simulink model "main_SLDV_2_2020"  (R2020b)
settings: Solver=FixedStepDiscrete  StartTime=0.0  StopTime=20.0  FixedStep=1  RelTol=1e-3
libraries: sldvlib x13, simulink x1
settings Model: Creator=ayj  LastModifiedBy=adije
settings DebuggingCC: UnconnectedInputMsg=none  UnconnectedOutputMsg=none  UnconnectedLineMsg=none  SFMachineParentedDataDiag=error
settings ConfigComp: DVMode=PropertyProving  DVTestSuiteOptimization=Auto  DVDetectOutOfBounds=on  DVProvingStrategy=FindViolation  DVMaxViolationSteps=12

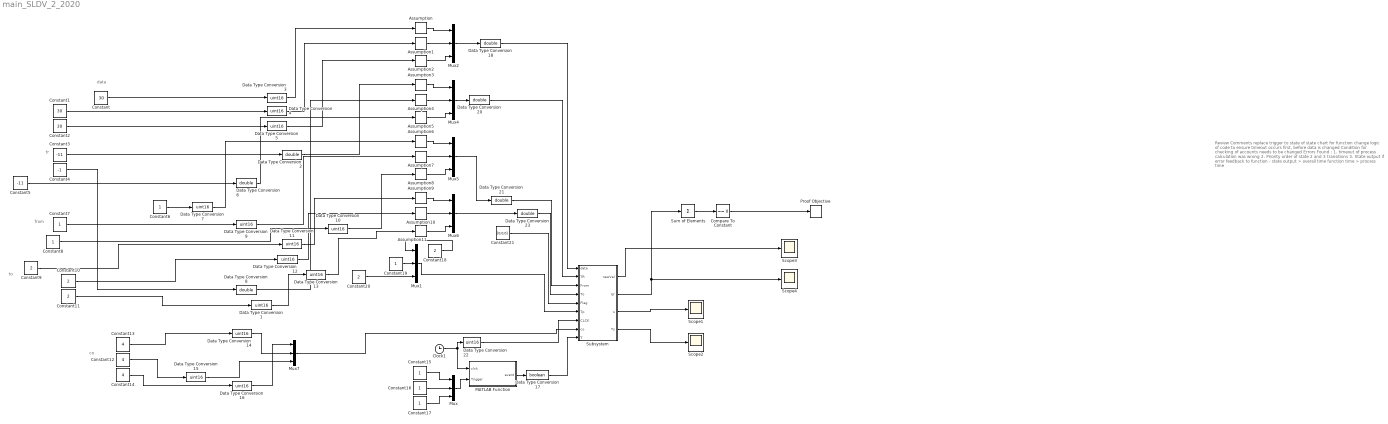
== system main_SLDV_2_2020 ==
  note: data
  note: tr
  note: from
  note: to
  note: co
  note: Review Comments
      | replace trigger to state of state chart for function
      | change logic of code to ensure timeout occurs first, before data is changed
      | Condition for checking of accounts needs to be changed
      |
      | Errors Found :
      | 1. timeout of process calculation was wrong
      | 2. Priority order of state 2 and 3 transitions
      | 3. State output if error feedback to function - state output > overall time
      | function time > process time
  Assumption : sldvlib/Objectives and Constraints/Assumption  enabled=on  customAVTBlockType=Assumption  intervals={30, 31, 32}  initial=off  dispValues=on  outEnabled=on
      settings: AttributesFormatString=%<intervals>  SourceProductBaseCode=SL
  Assumption1 : sldvlib/Objectives and Constraints/Assumption  enabled=on  customAVTBlockType=Assumption  intervals={30, 31, 32}  initial=off  dispValues=on  outEnabled=on
      settings: AttributesFormatString=%<intervals>  SourceProductBaseCode=SL
  Assumption{6..11} (6 alike) : sldvlib/Objectives and Constraints/Assumption  enabled=on  customAVTBlockType=Assumption  intervals={1,2,3}  initial=off  dispValues=on  outEnabled=on
      settings: AttributesFormatString=%<intervals>  SourceProductBaseCode=SL
  Assumption2 : sldvlib/Objectives and Constraints/Assumption  enabled=on  customAVTBlockType=Assumption  intervals={30, 31, 32}  initial=off  dispValues=on  outEnabled=on
      settings: AttributesFormatString=%<intervals>  SourceProductBaseCode=SL
  Assumption3 : sldvlib/Objectives and Constraints/Assumption  enabled=on  customAVTBlockType=Assumption  intervals={-10,+10,0, -11}  initial=off  dispValues=on  outEnabled=on
      settings: AttributesFormatString=%<intervals>  SourceProductBaseCode=SL
  Assumption4 : sldvlib/Objectives and Constraints/Assumption  enabled=on  customAVTBlockType=Assumption  intervals={-10,+10,0, -11}  initial=off  dispValues=on  outEnabled=on
      settings: AttributesFormatString=%<intervals>  SourceProductBaseCode=SL
  Assumption5 : sldvlib/Objectives and Constraints/Assumption  enabled=on  customAVTBlockType=Assumption  intervals={-10,+10,0, -11}  initial=off  dispValues=on  outEnabled=on
      settings: AttributesFormatString=%<intervals>  SourceProductBaseCode=SL
  Clock1 : Clock
  Compare To Constant : simulink/Logic and Bit Operations/Compare To Constant  relop===  const=0  OutDataTypeStr=boolean
  Constant : Constant  Value=30
  Constant1 : Constant  Value=30
  Constant{9..11,18,20} (5 alike) : Constant  Value=2
  Constant12 : Constant  Value=4
  Constant13 : Constant  Value=4
  Constant14 : Constant  Value=4
  Constant{6..8,15..17,19} (7 alike) : Constant
  Constant2 : Constant  Value=30
  Constant21 : Constant  Value=[0,0,0]
  Constant3 : Constant  Value=-11
  Constant4 : Constant  Value=-1
  Constant5 : Constant  Value=-11
  Data Type Conversion{1,3..5,7,9..16,22} (14 alike) : DataTypeConversion  OutDataTypeStr=uint16  RndMeth=Round
  Data Type Conversion17 : DataTypeConversion  OutDataTypeStr=boolean  RndMeth=Round
  Data Type Conversion{2,6,8,18,20..21,23} (7 alike) : DataTypeConversion  OutDataTypeStr=double  RndMeth=Round
  MATLAB Function : MATLAB Function  TreatAsAtomicUnit=on
  Mux{,1..2,4..7} (7 alike) : Mux  Inputs=3
  Proof Objective : sldvlib/Objectives and Constraints/Proof Objective  enabled=on  customAVTBlockType=Proof Objective  intervals=true  dispValues=on  outEnabled=off  enableStopSim=off
      settings: AttributesFormatString=%<intervals>  SourceProductBaseCode=SL
  Scope{1..4} (4 alike) : Scope
  Subsystem : Subsystem
  Sum of Elements : Sum  Inputs=+
  wires:
  Constant/1 -> Data Type Conversion3/1
  Constant1/1 -> Data Type Conversion4/1
  Constant2/1 -> Data Type Conversion5/1
  Constant3/1 -> Data Type Conversion2/1
  Constant6/1 -> Data Type Conversion7/1
  Constant7/1 -> Data Type Conversion9/1
  Constant8/1 -> Data Type Conversion10/1
  Constant9/1 -> Data Type Conversion11/1
  Constant10/1 -> Data Type Conversion12/1
  Constant11/1 -> Data Type Conversion1/1
  Constant4/1 -> Data Type Conversion8/1
  Constant5/1 -> Data Type Conversion6/1
  Constant13/1 -> Data Type Conversion14/1
  Constant12/1 -> Data Type Conversion15/1
  Constant14/1 -> Data Type Conversion16/1
  Data Type Conversion1/1 -> Data Type Conversion13/1
  Constant18/1 -> Mux1/1
  Constant20/1 -> Mux1/3
  Assumption4/1 -> Mux4/2
  Assumption7/1 -> Mux5/2
  Sum of Elements/1 -> Compare To Constant/1
  Data Type Conversion12/1 -> Assumption10/1
  Assumption/1 -> Mux2/1
  Mux6/1 -> Data Type Conversion23/1
  Assumption6/1 -> Mux5/1
  Assumption3/1 -> Mux4/1
  Data Type Conversion8/1 -> Assumption4/1
  Data Type Conversion9/1 -> Assumption7/1
  Assumption11/1 -> Mux6/3
  Data Type Conversion13/1 -> Assumption11/1
  Assumption1/1 -> Mux2/2
  Constant17/1 -> Mux/3
  Data Type Conversion11/1 -> Assumption9/1
  Data Type Conversion3/1 -> Assumption/1
  Data Type Conversion4/1 -> Assumption1/1
  Data Type Conversion2/1 -> Assumption3/1
  Mux5/1 -> Data Type Conversion21/1
  Constant15/1 -> Mux/1
  Compare To Constant/1 -> Proof Objective/1
  Mux2/1 -> Data Type Conversion18/1
  Assumption8/1 -> Mux5/3
  Data Type Conversion5/1 -> Assumption2/1
  Assumption9/1 -> Mux6/1
  MATLAB Function/1(event) -> Data Type Conversion17/1
  Data Type Conversion10/1 -> Assumption8/1
  Assumption10/1 -> Mux6/2
  Mux4/1 -> Data Type Conversion20/1
  Constant16/1 -> Mux/2
  Constant19/1 -> Mux1/2
  Assumption2/1 -> Mux2/3
  Assumption5/1 -> Mux4/3
  Data Type Conversion7/1 -> Assumption6/1
  Mux/1 -> MATLAB Function/2(Trigger)
  Clock1/1 -> Data Type Conversion22/1, MATLAB Function/1(clck)
  Data Type Conversion6/1 -> Assumption5/1
  Data Type Conversion16/1 -> Mux7/1
  Data Type Conversion14/1 -> Mux7/2
  Data Type Conversion15/1 -> Mux7/3
  Subsystem/2(Er) -> Sum of Elements/1, Scope4/1
  Data Type Conversion18/1 -> Subsystem/1(data)
  Data Type Conversion20/1 -> Subsystem/2(TR)
  Data Type Conversion21/1 -> Subsystem/3(From)
  Data Type Conversion23/1 -> Subsystem/4(To)
  Constant21/1 -> Subsystem/5(Flag)
  Mux1/1 -> Subsystem/6(Tp)
  Data Type Conversion22/1 -> Subsystem/7(CLCK)
  Mux7/1 -> Subsystem/8(co)
  Data Type Conversion17/1 -> Subsystem/9(T)
  Subsystem/1(newVal) -> Scope3/1
  Subsystem/3(s) -> Scope1/1
  Subsystem/4(Ts) -> Scope2/1

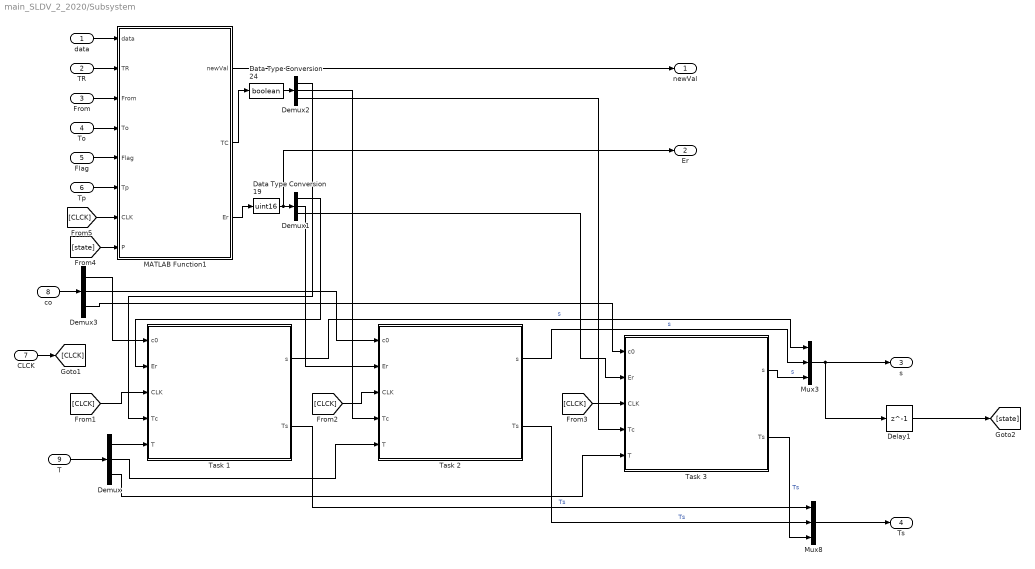
== system main_SLDV_2_2020/Subsystem ==
  data : Inport
  TR : Inport  Port=2
  From : Inport  Port=3
  To : Inport  Port=4
  Flag : Inport  Port=5
  Tp : Inport  Port=6
  CLCK : Inport  Port=7
  co : Inport  Port=8
  T : Inport  Port=9
  Data Type Conversion19 : DataTypeConversion  OutDataTypeStr=uint16  RndMeth=Round
  Data Type Conversion24 : DataTypeConversion  OutDataTypeStr=boolean  RndMeth=Round
  Delay1 : Delay  DelayLength=1
  Demux{,1..3} (4 alike) : Demux  Outputs=3
  MATLAB Function1 : MATLAB Function  TreatAsAtomicUnit=on
  Mux3 : Mux  Inputs=3
  Mux8 : Mux  Inputs=3
  Task 1 : Stateflow chart  TreatAsAtomicUnit=on
  Task 2 : Stateflow chart  TreatAsAtomicUnit=on
  Task 3 : Stateflow chart  TreatAsAtomicUnit=on
  newVal : Outport
  Er : Outport  Port=2
  s : Outport  Port=3
  Ts : Outport  Port=4
  wires:
  data/1 -> MATLAB Function1/1(data)
  Demux/2 -> Task 2/5(T)
  Demux1/2 -> Task 2/2(Er)
  Mux3/1 -> Delay1/1, s/1
  MATLAB Function1/1(newVal) -> newVal/1
  Demux1/3 -> Task 3/2(Er)
  [CLCK] -> MATLAB Function1/7(CLK)
  Task 2/1(s) -> Mux3/2  "s"
  Mux8/1 -> Ts/1
  Demux3/2 -> Task 2/1(c0)
  [CLCK] -> Task 3/3(CLK)
  Data Type Conversion19/1 -> Er/1, Demux1/1
  Task 1/1(s) -> Mux3/1  "s"
  To/1 -> MATLAB Function1/4(To)
  Demux2/1 -> Task 1/4(Tc)
  [CLCK] -> Task 1/3(CLK)
  Demux2/3 -> Task 3/4(Tc)
  Demux/1 -> Task 1/5(T)
  [CLCK] -> Task 2/3(CLK)
  Flag/1 -> MATLAB Function1/5(Flag)
  Demux3/1 -> Task 1/1(c0)
  Demux3/3 -> Task 3/1(c0)
  Demux2/2 -> Task 2/4(Tc)
  Task 3/2(Ts) -> Mux8/3  "Ts"
  Delay1/1 -> [state]
  Demux/3 -> Task 3/5(T)
  MATLAB Function1/3(Er) -> Data Type Conversion19/1
  MATLAB Function1/2(TC) -> Data Type Conversion24/1
  co/1 -> Demux3/1
  Demux1/1 -> Task 1/2(Er)
  Task 3/1(s) -> Mux3/3  "s"
  Tp/1 -> MATLAB Function1/6(Tp)
  Task 2/2(Ts) -> Mux8/2  "Ts"
  From/1 -> MATLAB Function1/3(From)
  CLCK/1 -> [CLCK]
  Task 1/2(Ts) -> Mux8/1  "Ts"
  [state] -> MATLAB Function1/8(P)
  Data Type Conversion24/1 -> Demux2/1
  T/1 -> Demux/1
  TR/1 -> MATLAB Function1/2(TR)

== stateflow chart main_SLDV_2_2020/Subsystem/Task 3 ==
  state Transact
    en:
    s = 1
    Ts = CLK
    du:
    c = c+1
  state Idle
    en:
    c = 0
    s = 0
    Ts = 0
  state Error
    en:
    s = 2
  state Error1
    en:
    s = 3
  Transact -> Error [order 2] : [c>=c0 || Er > 0]
  (default) -> Idle
  Idle -> Transact : [T==1]
  Transact -> Error1 [order 1] : [Tc == 1]
  Error -> Error1
  Error1 -> Idle
  data: c0 input uint16; Er input uint16; CLK input uint16; s output uint16; c local uint16; Ts output uint16; Tc input boolean; T input boolean

== matlab function main_SLDV_2_2020/Subsystem/MATLAB Function1 ==
  data: newVal output; data input double; TR input double; From input double; TC output; To input double; Flag input; Tp input; CLK input; P input; Er output
function [newVal, TC, Er] = fcn(data, TR, From, To, Flag, Tp, CLK, P)
persistent d
persistent f
persistent TC1
persistent Er1
persistent timeo
persistent init
persistent From1
persistent To1
persistent TR1
if(isempty(From1))
    From1 = [1;1;1];
end
if(isempty(To1))
    To1 = [1;1;1];
end
if(isempty(TR1))
    TR1 = [1;1;1];
end
if(isempty(d))
    d = [0;0;0];
end
if(isempty(init))
    init = 0;
end
if(isempty(f))
    f = [0;0;0];
end
if(isempty(TC1))
    TC1 = [0;0;0];
end
if(isempty(Er1))
    Er1 = [0;0;0];
end
if(isempty(timeo))
    timeo = [10,10,10];
end
if(init == 0)
    From1 = From;
    To1 = To;
    TR1 = TR;
    d = data;
    init = 1;
    f = Flag;
end


for i = 1:3
    if P(i) == 1
        if (f(From1(i)) == 0 && f(To1(i)) == 0)
            f(From1(i)) = 1;
            f(To1(i)) = 1;
            timeo(i) = CLK + Tp(i);
            if(d(From1(i)) + TR1(i) < 0 || d(To1(i)) - TR1(i) < 0)
                Er1(i) = 2;
                timeo(i) = 0;
            end
        end
        if CLK >= timeo(i)
            if(Er1(i) ~= 2)
                d(From1(i)) = d(From1(i)) + TR1(i);
                d(To1(i)) = d(To1(i)) - TR1(i);
                TC1(i) = 1;
            end
            f(From1(i)) = 0;
            f(To1(i)) = 0;
        end
    elseif P(i) == 2
        Er1(i) = 1;
    end
end

TC = TC1;
Er = Er1;
newVal = d;

== stateflow chart main_SLDV_2_2020/Subsystem/Task 2 ==
  state Transact
    en:
    s = 1
    Ts = CLK
    du:
    c = c+1
  state Idle
    en:
    c = 0
    s = 0
    Ts = 0
  state Error
    en:
    s = 2
  state Error1
    en:
    s = 3
  Transact -> Error [order 2] : [c>=c0 || Er > 0]
  Idle -> Transact : [T==1]
  (default) -> Idle
  Transact -> Error1 [order 1] : [Tc == 1]
  Error -> Error1
  Error1 -> Idle
  data: c0 input uint16; Er input uint16; CLK input uint16; s output uint16; c local uint16; Ts output uint16; Tc input boolean; T input boolean

== matlab function main_SLDV_2_2020/MATLAB Function ==
  data: clck input; event output; Trigger input
function event = fcn(clck, Trigger)
    event = clck==Trigger;

== stateflow chart main_SLDV_2_2020/Subsystem/Task 1 ==
  state Transact
    en:
    s = 1
    Ts = CLK
    du:
    c = c+1
  state Idle
    en:
    c = 0
    s = 0
    Ts = 0
  state Error
    en:
    s = 2
  state Error1
    en:
    s = 3
  Transact -> Error [order 2] : [c>=c0 || Er > 0]
  (default) -> Idle
  Idle -> Transact : [T==1]
  Transact -> Error1 [order 1] : [Tc == 1]
  Error -> Error1
  Error1 -> Idle
  data: c0 input uint16; Er input uint16; CLK input uint16; s output uint16; c local uint16; Ts output uint16; Tc input boolean; T input boolean
